simulink model "papersimulation_case2"  (R2024a)
settings: Solver=VariableStepAuto  StartTime=0.0  StopTime=10.0  RelTol=1e-3
settings Model: Creator=Administrator  LastModifiedBy=huchenglong
settings RTWCC: GPUComputeCapability=3.5

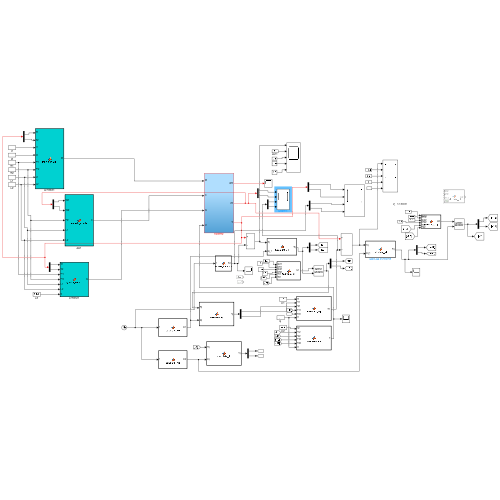
[thumbnail: Simulink's stored preview of the top-level diagram]
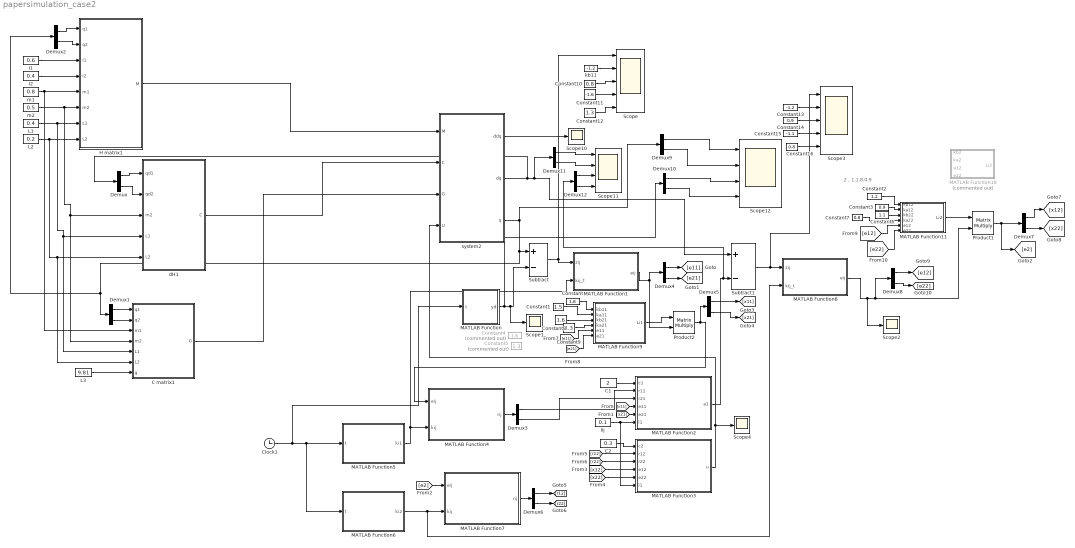
== system papersimulation_case2 ==
  note: 2，1,1.8.0.9
  C matrix1 : MATLAB Function  TreatAsAtomicUnit=on
  C1 : Constant  Value=2
  C2 : Constant  Value=0.3
  Clock1 : Clock
      settings: Decimation=30
  Constant : Constant  Value=1.8
  Constant1 : Constant  Value=1.5
  Constant10 : Constant  Value=0.8
  Constant11 : Constant  Value=-1.6
  Constant12 : Constant  Value=1.3
  Constant13 : Constant  Value=-1.2
  Constant14 : Constant  Value=0.9
  Constant15 : Constant  Value=-1.1
  Constant16 : Constant  Value=0.8
  Constant2 : Constant  Value=1.2
  Constant3 : Constant  Value=0.9
  Constant4 : Constant  Commented=on  Value=1.6
  Constant5 : Constant  Commented=on  Value=1.3
  Constant6 : Constant  Value=1.1
  Constant7 : Constant  Value=0.8
  Constant8 : Constant  Value=1.6
  Constant9 : Constant  Value=1.3
  Demux{,1..12} (13 alike) : Demux  Outputs=2
  H matrix1 : MATLAB Function  TreatAsAtomicUnit=on
  I1 : Constant  Value=0.6
  I2 : Constant  Value=0.4
  L1 : Constant  Value=0.4
  L2 : Constant  Value=0.2
  L3 : Constant  Value=9.81
  MATLAB Function : MATLAB Function  TreatAsAtomicUnit=on
  MATLAB Function1 : MATLAB Function  TreatAsAtomicUnit=on
  MATLAB Function10 : MATLAB Function  Commented=on  TreatAsAtomicUnit=on
  MATLAB Function11 : MATLAB Function  TreatAsAtomicUnit=on
  MATLAB Function2 : MATLAB Function  TreatAsAtomicUnit=on
  MATLAB Function3 : MATLAB Function  TreatAsAtomicUnit=on
  MATLAB Function4 : MATLAB Function  TreatAsAtomicUnit=on
  MATLAB Function5 : MATLAB Function  TreatAsAtomicUnit=on
  MATLAB Function6 : MATLAB Function  TreatAsAtomicUnit=on
  MATLAB Function7 : MATLAB Function  TreatAsAtomicUnit=on
  MATLAB Function8 : MATLAB Function  TreatAsAtomicUnit=on
  MATLAB Function9 : MATLAB Function  TreatAsAtomicUnit=on
  Product1 : Product  Multiplication=Matrix(*)  RndMeth=Zero
  Product2 : Product  Multiplication=Matrix(*)  RndMeth=Zero
  Scope : Scope  NumInputPorts=5
  Scope{1..2,4,10} (4 alike) : Scope
  Scope11 : Scope  NumInputPorts=4
  Scope12 : Scope  NumInputPorts=4
  Scope3 : Scope  NumInputPorts=5
  Subtract : Sum  Inputs=+-
  Subtract1 : Sum  Inputs=+-
  dH1 : MATLAB Function  TreatAsAtomicUnit=on
  kb11 : Constant  Value=-1.2
  lij : Constant  Value=0.1
  m1 : Constant  Value=0.8
  m2 : Constant  Value=0.5
  system2 : Subsystem
  wires:
  system2/3(q) -> Demux2/1, Demux1/1, Subtract/1, Demux9/1
  dH1/1(C) -> system2/2(C)
  MATLAB Function3/1(u) -> Scope4/1, system2/4(U)
  system2/1(ddq) -> Scope10/1
  C matrix1/1(G) -> system2/3(G)
  system2/2(dq) -> Demux/1, Demux11/1, Subtract1/1
  Clock1/1 -> MATLAB Function5/1(t), MATLAB Function6/1(t), MATLAB Function/1(t)
  MATLAB Function/1(yd) -> Demux10/1, Scope1/1, Subtract/2
  Subtract/1 -> Scope/1, MATLAB Function1/1(zij)
  lij/1 -> MATLAB Function2/6(l1), MATLAB Function3/6(l1)
  MATLAB Function5/1(ki1) -> MATLAB Function1/2(kij_t), MATLAB Function4/2(kij)
  MATLAB Function6/1(ki2) -> MATLAB Function8/2(kij_t), MATLAB Function7/2(kij)
  C1/1 -> MATLAB Function2/1(c1)
  MATLAB Function4/1(rij) -> Demux3/1
  C2/1 -> MATLAB Function3/1(c2)
  MATLAB Function2/1(a1) -> Demux12/1, Subtract1/2
  Subtract1/1 -> Scope3/1, MATLAB Function8/1(zij)
  L1/1 -> C matrix1/5(L1), dH1/4(L1), H matrix1/7(L1)
  m1/1 -> C matrix1/3(m1), H matrix1/5(m1)
  I1/1 -> H matrix1/3(I1)
  I2/1 -> H matrix1/4(I2)
  L2/1 -> C matrix1/6(L2), dH1/5(L2), H matrix1/8(L2)
  m2/1 -> C matrix1/4(m2), dH1/3(m2), H matrix1/6(m2)
  H matrix1/1(M) -> system2/1(M)
  L3/1 -> C matrix1/7(g)
  Demux/1 -> dH1/1(qd1)
  Demux/2 -> dH1/2(qd2)
  Demux1/1 -> C matrix1/1(q1)
  Demux1/2 -> C matrix1/2(q2)
  Demux2/1 -> H matrix1/1(q1)
  Demux2/2 -> H matrix1/2(q2)
  MATLAB Function1/1(eij) -> Demux4/1, Product2/2
  Demux3/1 -> MATLAB Function2/2(r11)
  Demux3/2 -> MATLAB Function2/3(r21)
  Demux4/1 -> [e11]
  [x11] -> MATLAB Function2/4(e11)
  [x21] -> MATLAB Function2/5(e21)
  Demux4/2 -> [e21]
  [x12] -> MATLAB Function3/4(e12)
  [x22] -> MATLAB Function3/5(e22)
  MATLAB Function7/1(rij) -> Demux6/1
  Demux6/1 -> [r12]
  Demux6/2 -> [r22]
  [r12] -> MATLAB Function3/2(r12)
  [r22] -> MATLAB Function3/3(r22)
  Constant/1 -> MATLAB Function9/1(kb11)
  Constant1/1 -> MATLAB Function9/2(ka11)
  [e21] -> MATLAB Function9/6(e21)
  MATLAB Function9/1(Li1) -> Product2/1
  Product2/1 -> Demux5/1, MATLAB Function4/1(eij)
  [e12] -> MATLAB Function11/5(e12)
  [e22] -> MATLAB Function11/6(e22)
  Constant2/1 -> MATLAB Function11/1(kb12)
  Constant3/1 -> MATLAB Function11/2(ka12)
  MATLAB Function11/1(Li2) -> Product1/1
  MATLAB Function8/1(eij) -> Scope2/1, Demux8/1, Product1/2
  Product1/1 -> [e2], Demux7/1
  Demux7/1 -> [x12]
  [e2] -> MATLAB Function7/1(eij)
  Demux5/1 -> [x11]
  Demux5/2 -> [x21]
  Demux7/2 -> [x22]
  Demux8/1 -> [e12]
  Demux8/2 -> [e22]
  Constant6/1 -> MATLAB Function11/3(kb22)
  Constant7/1 -> MATLAB Function11/4(ka22)
  Constant8/1 -> MATLAB Function9/3(kb21)
  Constant9/1 -> MATLAB Function9/4(ka21)
  Demux9/1 -> Scope12/1
  Demux9/2 -> Scope12/2
  Demux10/1 -> Scope12/3
  Demux10/2 -> Scope12/4
  Demux11/1 -> Scope11/1
  Demux11/2 -> Scope11/2
  Demux12/1 -> Scope11/3
  Demux12/2 -> Scope11/4
  kb11/1 -> Scope/2
  Constant10/1 -> Scope/3
  Constant11/1 -> Scope/4
  [e11] -> MATLAB Function9/5(e11)
  Constant12/1 -> Scope/5
  Constant13/1 -> Scope3/2
  Constant14/1 -> Scope3/3
  Constant15/1 -> Scope3/4
  Constant16/1 -> Scope3/5

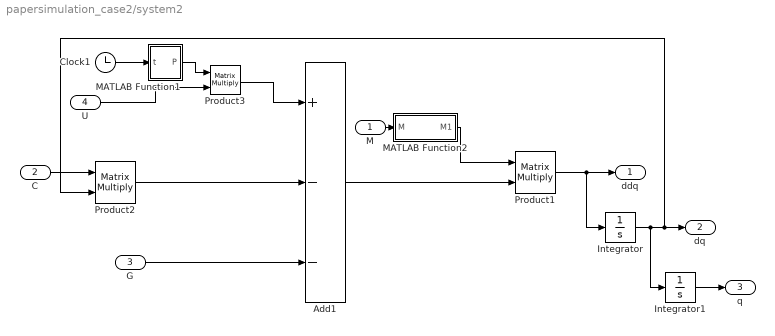
== system papersimulation_case2/system2 ==
  M : Inport
  C : Inport  Port=2
  G : Inport  Port=3
  U : Inport  Port=4
  Add1 : Sum  Inputs=+--
  Clock1 : Clock
      settings: Decimation=30
  Integrator : Integrator
  Integrator1 : Integrator  InitialCondition=[-1.2;1.9]
  MATLAB Function1 : MATLAB Function  TreatAsAtomicUnit=on
  MATLAB Function2 : MATLAB Function  TreatAsAtomicUnit=on
  Product1 : Product  Multiplication=Matrix(*)  RndMeth=Zero
  Product2 : Product  Multiplication=Matrix(*)  RndMeth=Zero
  Product3 : Product  Multiplication=Matrix(*)  RndMeth=Zero
  ddq : Outport
  dq : Outport  Port=2
  q : Outport  Port=3
  wires:
  G/1 -> Add1/3
  Add1/1 -> Product1/2
  M/1 -> MATLAB Function2/1(M)
  MATLAB Function2/1(M1) -> Product1/1
  Product1/1 -> Integrator/1, ddq/1
  Integrator/1 -> Integrator1/1, Product2/2, dq/1
  Integrator1/1 -> q/1
  C/1 -> Product2/1
  Product2/1 -> Add1/2
  Clock1/1 -> MATLAB Function1/1(t)
  MATLAB Function1/1(P) -> Product3/1
  U/1 -> Product3/2
  Product3/1 -> Add1/1

== matlab function papersimulation_case2/H matrix1 ==
  data: q1 input; q2 input; I1 input; M output; I2 input; m1 input; m2 input; L1 input; L2 input
function M = inertia_matrix(q1,q2,I1, I2, m1, m2, L1, L2)
    M11 = I1 + I2 + m1*(L1^2/4) + m2*(L1^2 + (L1^2/2) + L1*L2*cos(q2));
    M12 = I2 + m2*(L1^2/4 + (1/2)*L1*L2*cos(q2));
    M21 = M12;
    M22 = I2 + m2*(L2^2/4);
    M = [M11, M12; M21, M22];
end

== matlab function papersimulation_case2/dH1 ==
  data: qd1 input; qd2 input; C output; m2 input; L1 input; L2 input
function C = coriolis_matrix(qd1, qd2, m2, L1, L2)
    c = (1/2)*m2*L1*L2*sin(qd2);
    C11 = -c*qd2;
    C12 = -c*(qd1 + qd2);
    C21 = c*qd1;
    C22 = 0;
    C = [C11, C12; C21, C22];
end

== matlab function papersimulation_case2/MATLAB Function9 ==
  data: kb11 input; Li1 output; ka11 input; kb21 input; ka21 input; e11 input; e21 input
function Li1 = calculate_Lij(kb11, ka11,kb21,ka21,e11, e21)
    % 根据公式计算 Lij
    L11 = 1./((kb11 + e11).*(ka11 - e11));
    L21 = 1./((kb21 + e21).*(ka21 - e21));
    Li1 = diag([L11, L21]);
    
end

== matlab function papersimulation_case2/MATLAB Function10 ==
  data: kb2 input; Li2 output; ka2 input; e12 input; e22 input
function Li2 = calculate_Lij(kb2, ka2, e12, e22)
    % 根据公式计算 Lij
    L12 = 1./((kb2 + e12).*(ka2 - e12));
    L22 = 1./((kb2 + e22).*(ka2 - e22));
    Li2 = diag([L12, L22]);
    
end

== matlab function papersimulation_case2/MATLAB Function11 ==
  data: kb12 input; Li2 output; ka12 input; kb22 input; ka22 input; e12 input; e22 input
function Li2 = calculate_Lij(kb12, ka12,kb22, ka22, e12, e22)
    % 根据公式计算 Lij
    L12 = 1./((kb12 + e12).*(ka12 - e12));
    L22 = 1./((kb22 + e22).*(ka22 - e22));
    Li2 = diag([L12, L22]);
    
end

== matlab function papersimulation_case2/MATLAB Function1 ==
  data: zij input; eij output; kij_t input
function eij = calculate_eij(zij, kij_t)
    % 确保z为向量或标量形式
    % 根据公式计算eij
    eij = (1./kij_t).* atan(zij);
end

== matlab function papersimulation_case2/system2/MATLAB Function1 ==
  data: P output; t input
function P = P_t(t)
% 函数功能：计算时变矩阵P(t)
% 输入参数：
%   t - 时间变量
% 输出参数：
%   P - 时变矩阵

P = [0.6 + 0.1*sin(t), 0;
     0, 0.4 + 0.1*cos(t)];
end

== matlab function papersimulation_case2/system2/MATLAB Function2 ==
  data: M1 output; M input
function M1 = fcn(M)
%#codegen


M1 = inv(M);

== matlab function papersimulation_case2/MATLAB Function ==
  data: t input; yd output
function yd = desired_trajectory(t)
    % 计算期望轨迹的第一个元素
    yd_1 = 0.5 * sin(t);
    % 计算期望轨迹的第二个元
    yd_2 = 0.8 * cos(t);
    % 将两个元素组合成向量作为函数输出
    yd = [yd_1; yd_2];
end

== matlab function papersimulation_case2/MATLAB Function2 ==
  data: c1 input; r11 input; a1 output; r21 input; e11 input; e21 input; l1 input
function a1 = calculate_aij(c1,r11, r21, e11, e21,l1)
    % 计算 rij 和 tan(eij) 的乘积
    a11 = -c1 * (sqrt(abs(r11 * tan(e11))^2 + l1)) * r11 * tan(e11);
    a21 = -c1 * (sqrt(abs(r21 * tan(e21))^2 + l1)) * r21 * tan(e21);
    a1 =[a11; a21];
end

== matlab function papersimulation_case2/MATLAB Function3 ==
  data: c2 input; u output; r12 input; r22 input; e12 input; e22 input; l1 input
function u = calculate_aij(c2,r12, r22, e12, e22,l1)
    % 计算 rij 和 tan(eij) 的乘积
    a12 = -c2 * (sqrt(abs(r12 * tan(e12))^2 + l1)) * r12 * tan(e12);
    a22 = -c2 * (sqrt(abs(r22 * tan(e22))^2 + l1)) * r22 * tan(e22);
    
    u =[a12; a22];
end

== matlab function papersimulation_case2/MATLAB Function4 ==
  data: eij input; kij input; rij output
function rij = calculate_rij(eij, kij)
    % 确保 eij 和 kij 为向量或标量形式
    % 根据公式计算 rij
    rij = (cos(eij).^(-2)).* (kij.^(-1)).* (1 + tan(kij.* eij).^2).^(-1);
    % 确保 rij 大于0，若有小于0的值可进行修正等处理（这里简单取绝对值）
    rij = abs(rij); 
end

== matlab function papersimulation_case2/MATLAB Function5 ==
  data: t input; ki1 output
function ki1 = calculate_ki1(t)
    ki1 = (1 - 0.05)*exp(-3*t) + 0.05;
end

== matlab function papersimulation_case2/MATLAB Function6 ==
  data: t input; ki2 output
function ki2 = calculate_ki2(t)
    ki2 = (1 - 0.1)*exp(-2*t) + 0.1;
end

== matlab function papersimulation_case2/MATLAB Function7 ==
  data: eij input; kij input; rij output
function rij = calculate_rij(eij, kij)
    % 确保 eij 和 kij 为向量或标量形式
    % 根据公式计算 rij
    rij = (cos(eij).^(-2)).* (kij.^(-1)).* (1 + tan(kij.* eij).^2).^(-1);
    % 确保 rij 大于0，若有小于0的值可进行修正等处理（这里简单取绝对值）
    rij = abs(rij); 
end

== matlab function papersimulation_case2/MATLAB Function8 ==
  data: zij input; eij output; kij_t input
function eij = calculate_eij(zij, kij_t)
    % 确保z为向量或标量形式
    % 根据公式计算eij
    eij = (1./kij_t).* atan(zij);
end

== matlab function papersimulation_case2/C matrix1 ==
  data: q1 input; q2 input; G output; m1 input; m2 input; L1 input; L2 input; g input
function G = gravity_vector(q1,q2,m1, m2, L1, L2, g)
   
    G1 = (1/2)*m1*g*L1*cos(q1) + m2*g*((L2/2) + L1*cos(q1));
    G2 = (1/2)*m2*g*L2*cos(q1 + q2);
    G = [G1; G2];
end
